simulink model "lab1ex2"  (R2024a)
settings: Solver=VariableStepAuto  StartTime=0.0  StopTime=50  MaxStep=0.1  RelTol=1e-3
libraries: dspfdesign x1

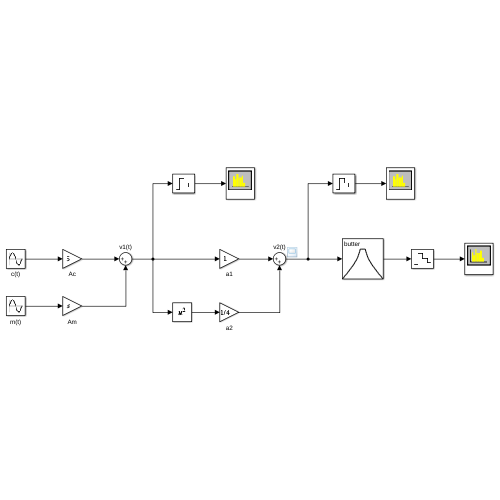
[thumbnail: Simulink's stored preview of the top-level diagram]
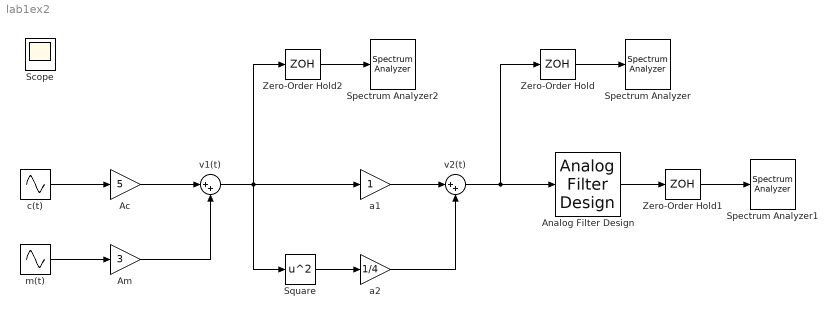
== system lab1ex2 ==
  Ac : Gain  Gain=5
  Am : Gain  Gain=3
  Analog Filter Design : dspfdesign/Analog Filter Design  method=Butterworth  filttype=Bandpass  N=8  Wlo=2*pi*15  Whi=2*pi*25  Rp=2  Rs=40
  Spectrum Analyzer : SpectrumAnalyzer  WindowPosition=[-20.000000,50.000000,800.000000,500.000000,]  ScopeFrameLocation=window  PlotAsTwoSidedSpectrum=off  SpectrumUnits=Watts  YLimits=[-2.25886471,20.32981977]
  Spectrum Analyzer1 : SpectrumAnalyzer  WindowPosition=[560.000000,350.000000,800.000000,500.000000,]  ScopeFrameLocation=window  PlotAsTwoSidedSpectrum=off  SpectrumUnits=Watts  YLimits=[-2.25886471,20.32981977]
  Spectrum Analyzer2 : SpectrumAnalyzer  WindowPosition=[560.000000,350.000000,800.000000,500.000000,]  ScopeFrameLocation=window  PlotAsTwoSidedSpectrum=off  SpectrumUnits=Watts  YLimits=[-2.25886471,20.32981977]
  Square : Math  Operator=square
  Zero-Order Hold : ZeroOrderHold  SampleTime=1/100
  Zero-Order Hold1 : ZeroOrderHold  SampleTime=1/100
  Zero-Order Hold2 : ZeroOrderHold  SampleTime=1/100
  a1 : Gain
  a2 : Gain  Gain=1/4
  c(t) : Sin  Frequency=2*pi*20  Phase=pi/2  SampleTime=0
  m(t) : Sin  Frequency=2*pi*4  Phase=pi/2  SampleTime=0
  v1(t) : Sum  Inputs=|++
  v2(t) : Sum  Inputs=|++
  Scope : Scope
  wires:
  m(t)/1 -> Am/1
  c(t)/1 -> Ac/1
  Ac/1 -> v1(t)/1
  v1(t)/1 -> Zero-Order Hold2/1, a1/1, Square/1
  a1/1 -> v2(t)/1
  a2/1 -> v2(t)/2
  Am/1 -> v1(t)/2
  v2(t)/1 -> Analog Filter Design/1, Zero-Order Hold/1
  Square/1 -> a2/1
  Zero-Order Hold/1 -> Spectrum Analyzer/1
  Zero-Order Hold1/1 -> Spectrum Analyzer1/1
  Analog Filter Design/1 -> Zero-Order Hold1/1
  Zero-Order Hold2/1 -> Spectrum Analyzer2/1
